simulink model "sampleModel1423"  (R2023a)
settings: Solver=VariableStepAuto  StartTime=0.0  StopTime=10.0  RelTol=1e-3
libraries: simulink x4, hdlsllib x2
settings Model: Creator=user1  LastModifiedBy=user1

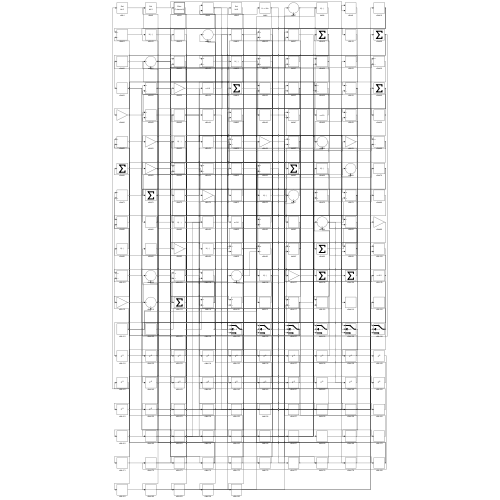
[thumbnail: Simulink's stored preview of the top-level diagram]
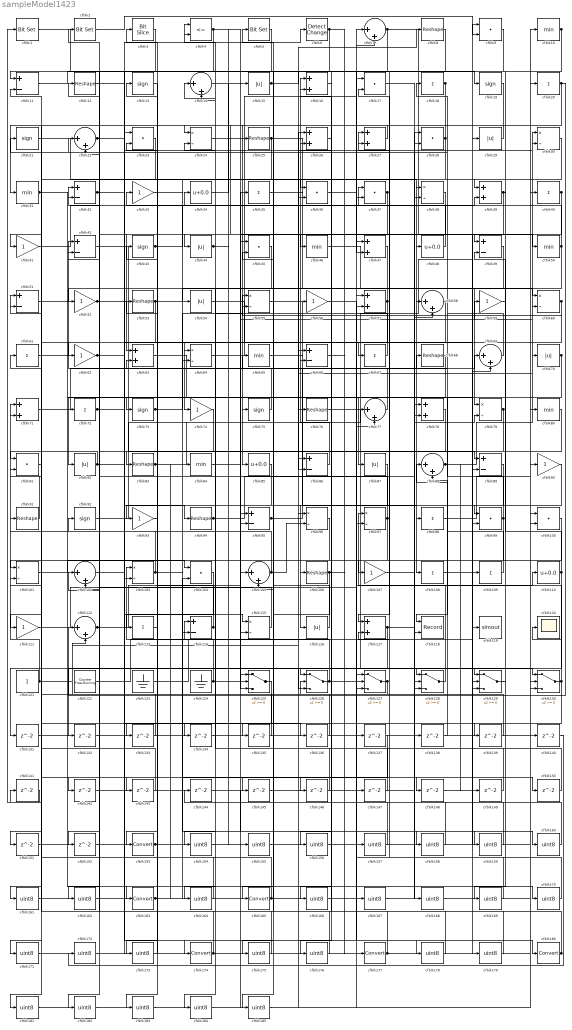
== system sampleModel1423 ==
  cfblk1 : simulink/Logic and Bit Operations/Bit Set  iBit=0
      settings: LibrarySourceBlock=|
      | hdlsllib/Logic and Bit
      | Operations/Bit Set
  cfblk{10,31,46,50,65,80,84} (7 alike) : MinMax
  cfblk{9,17,23,28,36..37,45,81,99..100,104} (11 alike) : DotProduct  OutDataTypeStr=Inherit: Inherit via internal rule
  cfblk{24,30,38,55,60,64,79,96..97,101,103,115} (12 alike) : Product  Inputs=*/  RndMeth=Zero  SaturateOnIntegerOverflow=on
  cfblk{7,14,22,58,69,77,88,102,105,112} (10 alike) : Sum  Inputs=|++
  cfblk{8,12,25,53,68,76,83,91,94,106} (10 alike) : Reshape
  cfblk{33,41,52,56,59,62,74,90,93,107,111} (11 alike) : Gain
  cfblk{18,20,35,40,61,67,72,98,108..109,113} (11 alike) : Sum  Inputs=+
  cfblk{11,32,42,49,51,66,86,89,95,114} (10 alike) : Sum  Inputs=+-
  cfblk{34,48,85,110} (4 alike) : Bias  Bias=0.0  SaturateOnIntegerOverflow=off
  cfblk{15,29,44,54,70,82,87,116} (8 alike) : Abs  SaturateOnIntegerOverflow=off
  cfblk{16,26..27,39,47,57,63,71,78,117} (10 alike) : Sum
  cfblk118 : Record  FileSettingsInternal="{\"entries\":[{\"content\":{\"excelSettings\":{\"content\":{},\"type\":\"Streamout.ExcelSettings\"}},\"type\":\"Streamout.FileSettingStorage\",\"uuid\":\"\"}],\"packageUris\":[\"http:\\/\\/schema.mathworks.com\\/mf0\\/streamout_blocks\\/R2020a\"],\"version\":\"1.0\"}"  Layout=[1 1]  SignalsInternal="{\"entries\":[{\"content\":{\"signals\":[{\"content\":{\"blockPath\":[],\"dimensions\":[1],\"domain\":\"\",\"lineColor\":\"#a2142f\",\"plots\":[1],\"port\":1,\"sid\":[\"\"],\"signalID\":379,\"signalName\":\"cfblk70\"},\"type\":\"RecordBlkView.Signal\",\"uuid\":\"\"},{\"content\":{\"blockPath\":[],\"dimensions\":[1],\"domain\":\"\",\"lineColor\":\"#139fff\",\"plots\":[1],\"port\":2,\"sid\":[\"\"],\"signalID\":383,\"signalName\":\"cfblk89\"},\"type\":\"RecordBlkView.Signal\",\"uuid\":\"\"}]},\"type\":\"RecordBlkView.InputSignals\",\"uuid\":\"\"}],\"packageUris\":[\"http:\\/\\/schema.mathworks.com\\/mf0\\/streamout_blocks\\/R2020a\"],\"version\":\"1.0\"}"  VisualizationBindings="{\"xyplotplugin\":{\"info\":[{\"series\":[{\"bindingParametersList\":[{\"parameter\":\"X-Axis\",\"signalID\":379,\"signalName\":\"cfblk70\"},{\"parameter\":\"Y-Axis\",\"signalID\":383,\"signalName\":\"cfblk89\"}],\"seriesID\":8776}],\"subplotID\":1}]}}"  CompatibilityTag=XY  st=-1
  cfblk119 : ToWorkspace  VariableName=simout  SaveFormat=Timeseries  SampleTime=-1
  cfblk120 : Scope
  cfblk121 : Constant  SampleTime=-1
  cfblk122 : hdlsllib/Sources/Counter Free-Running  NumBits=16  tsamp=-1
  cfblk123 : Ground
  cfblk124 : Ground
  cfblk{125..130} (6 alike) : Switch  SaturateOnIntegerOverflow=off  InputSameDT=off
  cfblk{13,19,21,43,73,75,92} (7 alike) : Signum
  cfblk{131..152} (22 alike) : Delay  SampleTime=1
  cfblk{153,163,165,174,177,180} (6 alike) : DataTypeConversion  SaturateOnIntegerOverflow=off  RndMeth=Floor
  cfblk{154..162,164,166..173,175..176,178..179,181..185} (27 alike) : DataTypeConversion  OutDataTypeStr=uint8  SaturateOnIntegerOverflow=off  RndMeth=Floor
  cfblk2 : simulink/Logic and Bit Operations/Bit Set  iBit=0
      settings: LibrarySourceBlock=|
      | hdlsllib/Logic and Bit
      | Operations/Bit Set
  cfblk3 : hdlsllib/Logic and Bit Operations/Bit Slice  lidx=7  ridx=0
  cfblk4 : RelationalOperator  Operator=<=  OutDataTypeStr=boolean  InputSameDT=off
  cfblk5 : simulink/Logic and Bit Operations/Bit Set  iBit=0
      settings: LibrarySourceBlock=|
      | hdlsllib/Logic and Bit
      | Operations/Bit Set
  cfblk6 : simulink/Logic and Bit Operations/Detect Change  vinit=0  OutDataTypeStr=boolean
      settings: LibrarySourceBlock=|
      | hdlsllib/Logic and Bit
      | Operations/Detect
      | Change
  wires:
  cfblk34/1 -> cfblk15/1
  cfblk124/1 -> cfblk103/1, cfblk126/1
  cfblk58/1 -> cfblk74/1
  cfblk76/1 -> cfblk130/1
  cfblk25/1 -> cfblk79/1, cfblk64/2
  cfblk88/1 -> cfblk30/1, cfblk149/1
  cfblk41/1 -> cfblk34/1
  cfblk113/1 -> cfblk33/1
  cfblk121/1 -> cfblk71/1, cfblk36/2, cfblk128/1
  cfblk61/1 -> cfblk163/1
  cfblk96/1 -> cfblk101/1
  cfblk27/1 -> cfblk44/1
  cfblk117/1 -> cfblk59/1, cfblk131/1, cfblk132/1
  cfblk68/1 -> cfblk82/1
  cfblk97/1 -> cfblk32/1, cfblk27/2, cfblk146/1
  cfblk3/1 -> cfblk11/1
  cfblk86/1 -> cfblk16/1
  cfblk28/1 -> cfblk108/1, cfblk25/1
  cfblk75/1 -> cfblk42/1
  cfblk91/1 -> cfblk71/2
  cfblk38/1 -> cfblk62/1
  cfblk64/1 -> cfblk7/1
  cfblk63/1 -> cfblk87/1
  cfblk10/1 -> cfblk117/1, cfblk49/1, cfblk95/2
  cfblk42/1 -> cfblk89/1
  cfblk50/1 -> cfblk13/1, cfblk134/1
  cfblk15/1 -> cfblk8/1, cfblk185/1
  cfblk95/1 -> cfblk69/1, cfblk70/1
  cfblk18/1 -> cfblk31/1, cfblk151/1
  cfblk100/1 -> cfblk153/1
  cfblk123/1 -> cfblk29/1
  cfblk87/1 -> cfblk116/1
  cfblk130/1 -> cfblk37/1, cfblk120/1, cfblk181/1
  cfblk128/1 -> cfblk97/1
  cfblk55/1 -> cfblk98/1
  cfblk37/1 -> cfblk63/1, cfblk86/2
  cfblk29/1 -> cfblk24/1
  cfblk57/1 -> cfblk52/1, cfblk113/1, cfblk162/1
  cfblk24/1 -> cfblk85/1
  cfblk40/1 -> cfblk129/2, cfblk139/1
  cfblk71/1 -> cfblk47/1
  cfblk112/1 -> cfblk12/1, cfblk60/2
  cfblk47/1 -> cfblk73/1
  cfblk82/1 -> cfblk81/1, cfblk94/1
  cfblk66/1 -> cfblk177/1
  cfblk56/1 -> cfblk180/1
  cfblk14/1 -> cfblk50/1
  cfblk30/1 -> cfblk41/1
  cfblk72/1 -> cfblk30/2, cfblk152/1
  cfblk22/1 -> cfblk38/2, cfblk6/1, cfblk178/1
  cfblk35/1 -> cfblk48/1
  cfblk46/1 -> cfblk119/1
  cfblk9/1 -> cfblk47/2
  cfblk8/1 -> cfblk46/1
  cfblk81/1 -> cfblk51/1
  cfblk31/1 -> cfblk126/3, cfblk170/1
  cfblk67/1 -> cfblk24/2
  cfblk70/1 -> cfblk118/1, cfblk127/3
  cfblk110/1 -> cfblk49/2, cfblk154/1
  cfblk126/1 -> cfblk114/1, cfblk110/1
  cfblk52/1 -> cfblk89/2, cfblk125/3
  cfblk99/1 -> cfblk65/1, cfblk115/2, cfblk127/2, cfblk18/1
  cfblk79/1 -> cfblk142/1, cfblk175/1
  cfblk21/1 -> cfblk125/1
  cfblk92/1 -> cfblk9/1
  cfblk98/1 -> cfblk40/1
  cfblk78/1 -> cfblk165/1
  cfblk69/1 -> cfblk21/1
  cfblk94/1 -> cfblk79/2, cfblk4/1
  cfblk1/1 -> cfblk76/1
  cfblk33/1 -> cfblk54/1
  cfblk111/1 -> cfblk7/2
  cfblk43/1 -> cfblk75/1, cfblk39/2, cfblk128/3
  cfblk83/1 -> cfblk68/1, cfblk148/1
  cfblk5/1 -> cfblk72/1
  cfblk12/1 -> cfblk36/1
  cfblk101/1 -> cfblk104/1
  cfblk7/1 -> cfblk69/2, cfblk176/1
  cfblk103/1 -> cfblk2/1, cfblk158/1
  cfblk116/1 -> cfblk22/1
  cfblk65/1 -> cfblk109/1
  cfblk114/1 -> cfblk53/1, cfblk43/1
  cfblk102/1 -> cfblk174/1
  cfblk59/1 -> cfblk99/1
  cfblk48/1 -> cfblk14/1
  cfblk62/1 -> cfblk115/1, cfblk64/1
  cfblk49/1 -> cfblk107/1
  cfblk20/1 -> cfblk112/1, cfblk106/1, cfblk39/1
  cfblk54/1 -> cfblk86/1
  cfblk106/1 -> cfblk145/1, cfblk167/1
  cfblk53/1 -> cfblk58/1, cfblk60/1, cfblk111/1
  cfblk85/1 -> cfblk93/1
  cfblk73/1 -> cfblk55/1, cfblk129/3
  cfblk122/1 -> cfblk97/2
  cfblk6/1 -> cfblk105/2, cfblk157/1
  cfblk89/1 -> cfblk118/2
  cfblk115/1 -> cfblk42/2
  cfblk60/1 -> cfblk55/2, cfblk164/1
  cfblk44/1 -> cfblk14/2, cfblk125/2
  cfblk105/1 -> cfblk91/1, cfblk96/2
  cfblk2/1 -> cfblk9/2
  cfblk77/1 -> cfblk32/2
  cfblk109/1 -> cfblk88/2
  cfblk4/1 -> cfblk103/2, cfblk67/1, cfblk155/1
  cfblk74/1 -> cfblk83/1
  cfblk45/1 -> cfblk114/2
  cfblk32/1 -> cfblk27/1, cfblk136/1
  cfblk11/1 -> cfblk19/1
  cfblk39/1 -> cfblk129/1, cfblk128/2
  cfblk51/1 -> cfblk77/1
  cfblk84/1 -> cfblk35/1
  cfblk127/1 -> cfblk112/2, cfblk126/2
  cfblk36/1 -> cfblk38/1
  cfblk131/1 -> cfblk130/2
  cfblk132/1 -> cfblk22/2
  cfblk13/1 -> cfblk133/1
  cfblk133/1 -> cfblk81/2
  cfblk134/1 -> cfblk77/2
  cfblk125/1 -> cfblk135/1
  cfblk135/1 -> cfblk63/2
  cfblk136/1 -> cfblk51/2
  cfblk138/1 -> cfblk88/1
  cfblk139/1 -> cfblk16/2
  cfblk141/1 -> cfblk1/1
  cfblk142/1 -> cfblk58/2
  cfblk19/1 -> cfblk143/1
  cfblk143/1 -> cfblk11/2
  cfblk145/1 -> cfblk37/2
  cfblk146/1 -> cfblk4/2
  cfblk147/1 -> cfblk45/2
  cfblk149/1 -> cfblk117/2
  cfblk107/1 -> cfblk150/1
  cfblk150/1 -> cfblk127/1
  cfblk151/1 -> cfblk99/2
  cfblk152/1 -> cfblk130/3
  cfblk153/1 -> cfblk20/1, cfblk3/1
  cfblk154/1 -> cfblk100/1
  cfblk155/1 -> cfblk100/2
  cfblk26/1 -> cfblk156/1
  cfblk156/1 -> cfblk57/2
  cfblk157/1 -> cfblk26/1
  cfblk158/1 -> cfblk26/2
  cfblk144/1 -> cfblk159/1
  cfblk159/1 -> cfblk28/1
  cfblk108/1 -> cfblk160/1
  cfblk160/1 -> cfblk144/1
  cfblk137/1 -> cfblk161/1
  cfblk161/1 -> cfblk104/2
  cfblk162/1 -> cfblk137/1
  cfblk163/1 -> cfblk28/2, cfblk84/1, cfblk105/1
  cfblk164/1 -> cfblk61/1
  cfblk165/1 -> cfblk138/1, cfblk92/1
  cfblk16/1 -> cfblk166/1
  cfblk166/1 -> cfblk78/1
  cfblk167/1 -> cfblk78/2
  cfblk17/1 -> cfblk168/1
  cfblk168/1 -> cfblk140/1
  cfblk129/1 -> cfblk169/1
  cfblk169/1 -> cfblk17/1
  cfblk170/1 -> cfblk17/2
  cfblk23/1 -> cfblk171/1
  cfblk171/1 -> cfblk57/1
  cfblk140/1 -> cfblk172/1
  cfblk172/1 -> cfblk23/1
  cfblk104/1 -> cfblk173/1
  cfblk173/1 -> cfblk23/2
  cfblk174/1 -> cfblk141/1, cfblk101/2
  cfblk175/1 -> cfblk102/1
  cfblk176/1 -> cfblk102/2
  cfblk177/1 -> cfblk96/1, cfblk10/1
  cfblk178/1 -> cfblk66/1
  cfblk148/1 -> cfblk179/1
  cfblk179/1 -> cfblk66/2
  cfblk180/1 -> cfblk95/1, cfblk5/1
  cfblk181/1 -> cfblk56/1
  cfblk80/1 -> cfblk182/1
  cfblk182/1 -> cfblk147/1
  cfblk93/1 -> cfblk183/1
  cfblk183/1 -> cfblk80/1
  cfblk90/1 -> cfblk184/1
  cfblk184/1 -> cfblk45/1
  cfblk185/1 -> cfblk90/1
